simulink model "ReactionWheelPendulum"  (R2019b)
settings: Solver=FixedStepDiscrete  StartTime=0.0  StopTime=1  FixedStep=.005  RelTol=1e-3
values from neighbouring files (symbols this model uses):
  Bb = 0.0    [ReactionWheelPendulum.sldd]
  BodyCGDist_mm = 73.103937    [ReactionWheelPendulum.sldd]
  g_mps_2 = 9.81    [ReactionWheelPendulum.sldd]
  GearRatio_na = 3.0    [ReactionWheelPendulum.sldd]
  IBodyPivot_kgm_2 = 0.004054322    [ReactionWheelPendulum.sldd]
  IWheelCG_kgm_2 = 0.00010714633    [ReactionWheelPendulum.sldd]
  IWheelPivot_kgm_2 = 0.00054580359    [ReactionWheelPendulum.sldd]
  MassBody_kg = 0.49436    [ReactionWheelPendulum.sldd]
  MassWheel_kg = 0.092779    [ReactionWheelPendulum.sldd]
  WheelCGDist_mm = 68.760176    [ReactionWheelPendulum.sldd]
undefined symbols (not defined in the file or in its folder): DiscIntNeverNeededParam
libraries: simulink x6, simulink_extras x3
settings Model: DataDictionary=ReactionWheelPendulum.sldd  Creator=aloehr  LastModifiedBy=aloehr

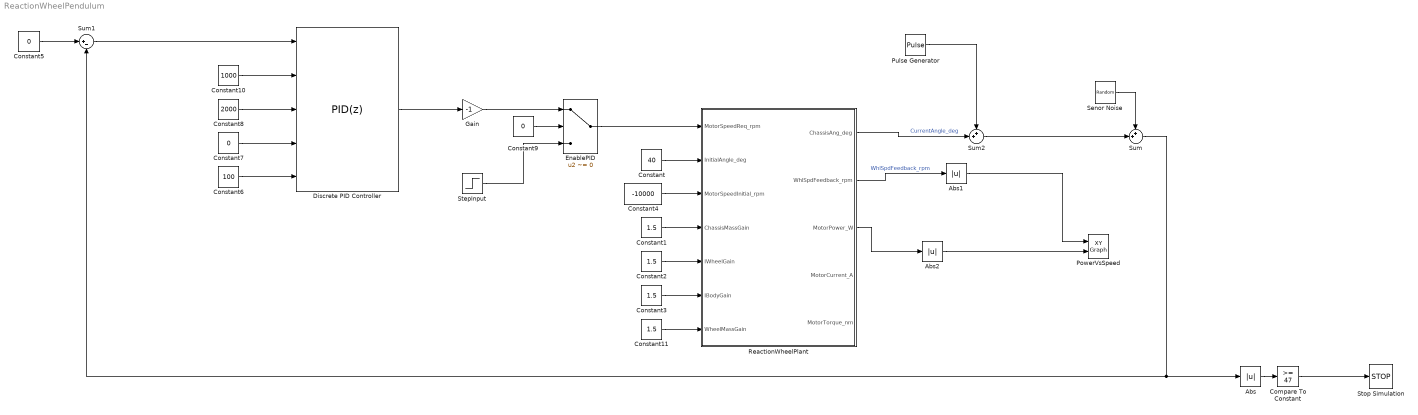
== system ReactionWheelPendulum ==
  Abs : Abs
  Abs1 : Abs
  Abs2 : Abs
  Compare To Constant : simulink/Logic and Bit Operations/Compare To Constant  relop=>=  const=47  OutDataTypeStr=boolean
  Constant : Constant  Value=40
  Constant{1..3,11} (4 alike) : Constant  Value=1.5
  Constant10 : Constant  Value=1000
  Constant4 : Constant  Value=-10000
  Constant5 : Constant  Value=0
  Constant6 : Constant  Value=100
  Constant7 : Constant  Value=0
  Constant8 : Constant  Value=2000
  Constant9 : Constant  Value=0
  Discrete PID Controller : simulink/Continuous/PID Controller  Controller=PID  Form=Parallel  TimeDomain=Discrete-time  SampleTime=-1  IntegratorMethod=Forward Euler  FilterMethod=Forward Euler  ControllerParametersSource=external  P=1  I=1  D=0  UseFilter=on  N=100  TunerSelectOption=Transfer Function Based (PID Tuner App)  InitialConditionSource=internal  InitialConditionForIntegrator=0  InitialConditionForFilter=0  DifferentiatorICPrevScaledInput=0  ExternalReset=none  TrackingMode=off  Kt=1  LimitOutput=on  UpperSaturationLimit=11000  LowerSaturationLimit=-11000  LinearizeAsGain=off  AntiWindupMode=none  Kb=1  POutMin=[]  POutMax=[]  IOutMin=[]  IOutMax=[]  DOutMin=[]  DOutMax=[]  NOutMin=[]  NOutMax=[]  SumOutMin=[]  SumOutMax=[]  SaturationOutMin=[]  SaturationOutMax=[]  PParamMin=[]  PParamMax=[]  IParamMin=[]  IParamMax=[]  DParamMin=[]  DParamMax=[]  NParamMin=[]  NParamMax=[]  KbParamMin=[]  KbParamMax=[]  KtParamMin=[]  KtParamMax=[]  KbOutMin=[]  KbOutMax=[]  KtOutMin=[]  KtOutMax=[]  IntegratorOutMin=[]  IntegratorOutMax=[]  FilterOutMin=[]  FilterOutMax=[]  SumI1OutMin=[]  SumI1OutMax=[]  SumI2OutMin=[]  SumI2OutMax=[]  SumI3OutMin=[]  SumI3OutMax=[]  SumI4OutMin=[]  SumI4OutMax=[]  SumDOutMin=[]  SumDOutMax=[]  DifferentiatorOutMin=[]  DifferentiatorOutMax=[]  FilterDiffOutCoefMin=[]  FilterDiffOutCoefMax=[]  ReciprocalOutMin=[]  ReciprocalOutMax=[]  SumDenOutMin=[]  SumDenOutMax=[]  SumNumOutMin=[]  SumNumOutMax=[]  DivideOutMin=[]  DivideOutMax=[]  IntegratorContinuousStateAttributes=''  IntegratorStateMustResolveToSignalObject=off  IntegratorRTWStateStorageClass=Auto  FilterContinuousStateAttributes=''  FilterStateMustResolveToSignalObject=off  FilterRTWStateStorageClass=Auto  ParallelPVariant=ExternalParameters  IdealPVariant=Disabled  IVariant=ExternalParameters  DVariant=ExternalParameters  IntegratorVariant=Discrete  SatVariant=Enabled  AWVariant=Passthrough  PCopyVariant=Disabled  TRVariant=Disabled  FdbkBlocksVariant=Forward  IdealPFdbkVariant=Disabled  SatFdbkVariant=Disabled  DerivativeFilterVariant=ForwardEulerFilter  NVariant=ExternalParameters  NCopyVariant=Disabled  FilterICVariant=InternalICsFilter  IntegratorICVariant=InternalICs  ExternalResetVariant=Disabled  TRSumVariant=Passthrough  SumFdbkVariant=Disabled  SumVariant=Sum_PID
  EnablePID : Switch  Criteria=u2 ~= 0
  Gain : Gain  Gain=-1
  PowerVsSpeed : simulink/Sinks/XY Graph  xmin=0  xmax=11000  ymin=0  ymax=300  st=-1
  Pulse Generator : DiscretePulseGenerator  PulseType=Time based  Amplitude=5  Period=3  PulseWidth=10  PhaseDelay=1
  ReactionWheelPlant : Subsystem
  Senor Noise : UniformRandomNumber  Minimum=-.1  Maximum=.1  SampleTime=0.1
  StepInput : Step  Time=.015  Before=-10000  After=11000  SampleTime=0
  Stop Simulation : Stop
  Sum : Sum  Inputs=++|
  Sum1 : Sum  Inputs=|+-
  Sum2 : Sum  Inputs=++|
  wires:
  Constant/1 -> ReactionWheelPlant/2(InitialAngle_deg)
  Constant1/1 -> ReactionWheelPlant/4(ChassisMassGain)
  Constant2/1 -> ReactionWheelPlant/5(IWheelGain)
  Constant3/1 -> ReactionWheelPlant/6(IBodyGain)
  Senor Noise/1 -> Sum/1
  Sum/1 -> Sum1/2, Abs/1
  Constant5/1 -> Sum1/1
  Sum1/1 -> Discrete PID Controller/1
  Discrete PID Controller/1 -> Gain/1
  Constant6/1 -> Discrete PID Controller/5
  Constant7/1 -> Discrete PID Controller/4
  Constant8/1 -> Discrete PID Controller/3
  Compare To Constant/1 -> Stop Simulation/1
  Constant10/1 -> Discrete PID Controller/2
  Gain/1 -> EnablePID/1
  EnablePID/1 -> ReactionWheelPlant/1(MotorSpeedReq_rpm)
  Abs/1 -> Compare To Constant/1
  ReactionWheelPlant/3(MotorPower_W) -> Abs2/1
  ReactionWheelPlant/2(WhlSpdFeedback_rpm) -> Abs1/1  "WhlSpdFeedback_rpm"
  Abs1/1 -> PowerVsSpeed/1
  Abs2/1 -> PowerVsSpeed/2
  Constant9/1 -> EnablePID/2
  StepInput/1 -> EnablePID/3
  ReactionWheelPlant/1(ChassisAng_deg) -> Sum2/2  "CurrentAngle_deg"
  Sum2/1 -> Sum/2
  Constant11/1 -> ReactionWheelPlant/7(WheelMassGain)
  Pulse Generator/1 -> Sum2/1
  Constant4/1 -> ReactionWheelPlant/3(MotorSpeedInitial_rpm)

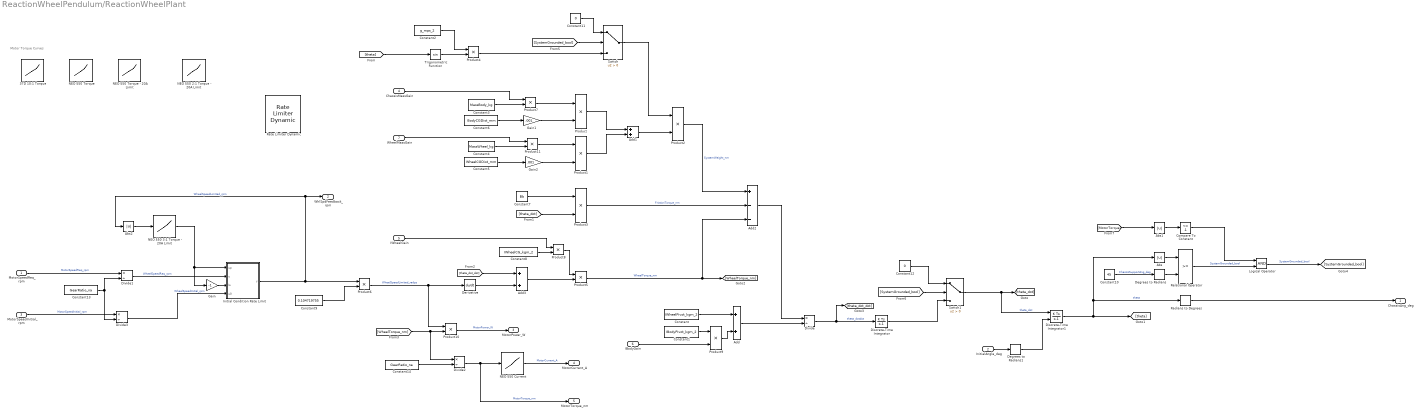
== system ReactionWheelPendulum/ReactionWheelPlant ==
  note: Motor Torque Curves
  MotorSpeedReq_rpm : Inport
  InitialAngle_deg : Inport  Port=2
  MotorSpeedInitial_rpm : Inport  Port=3
  ChassisMassGain : Inport  Port=4
  IWheelGain : Inport  Port=5
  IBodyGain : Inport  Port=6
  WheelMassGain : Inport  Port=7
  37D 10:1 Torque : Lookup_n-D  NumberOfTableDimensions=1  BreakpointsForDimension1=[0,1000]  Table=[55800,0.001]  InternalRulePriority=Speed  RndMeth=Simplest  InputSameDT=on
  Abs : Abs
  Abs1 : Abs
  Abs2 : Abs
  Add : Sum
  Add1 : Sum
  Add2 : Sum  Inputs=+--
  Add3 : Sum
  Compare To Constant : simulink/Logic and Bit Operations/Compare To Constant  relop=<=  const=.1  OutDataTypeStr=boolean
  Constant : Constant  Value=IWheelPivot_kgm_2  VectorParams1D=off
  Constant1 : Constant  Value=IBodyPivot_kgm_2
  Constant10 : Constant  Value=45
  Constant11 : Constant  Value=0
  Constant12 : Constant  Value=0
  Constant13 : Constant  Value=GearRatio_na
  Constant14 : Constant  Value=GearRatio_na
  Constant2 : Constant  Value=g_mps_2
  Constant3 : Constant  Value=MassBody_kg
  Constant4 : Constant  Value=MassWheel_kg
  Constant5 : Constant  Value=WheelCGDist_mm
  Constant6 : Constant  Value=BodyCGDist_mm
  Constant7 : Constant  Value=Bb
  Constant8 : Constant  Value=IWheelCG_kgm_2
  Constant9 : Constant  Value=0.104719755
  Degrees to Radians : simulink_extras/Transformations/Degrees to Radians
  Degrees to Radians1 : simulink_extras/Transformations/Degrees to Radians
  Derivative : Derivative
  Discrete-Time Integrator : DiscreteIntegrator  SampleTime=-1  ICPrevOutput=DiscIntNeverNeededParam  ICPrevScaledInput=DiscIntNeverNeededParam
  Discrete-Time Integrator1 : DiscreteIntegrator  InitialConditionSource=external  SampleTime=-1  ICPrevOutput=DiscIntNeverNeededParam  ICPrevScaledInput=DiscIntNeverNeededParam
  Divide{,1..3} (4 alike) : Product  Inputs=*/
  Gain : Gain  Gain=-1
  Gain1 : Gain  Gain=.001
  Gain2 : Gain  Gain=.001
  Initial Condition Rate Limit : Subsystem
  Logical Operator : Logic  AllPortsSameDT=off  OutDataTypeStr=boolean
  NEO 550 2:1 Torque - 20A Limit : Lookup_n-D  NumberOfTableDimensions=1  BreakpointsForDimension1=[0,4500,5500]  Table=[35000,35000,0]  InternalRulePriority=Speed  RndMeth=Simplest  InputSameDT=on
  NEO 550 3:1 Torque - 20A Limit : Lookup_n-D  NumberOfTableDimensions=1  BreakpointsForDimension1=[0,3000,3666.667]  Table=[35000,35000,0]  InternalRulePriority=Speed  RndMeth=Simplest  InputSameDT=on
  NEO 550 Current : Lookup_n-D  NumberOfTableDimensions=1  BreakpointsForDimension1=[0,.97]  Table=[0,100]  InternalRulePriority=Speed  RndMeth=Simplest  InputSameDT=on
  NEO 550 Torque : Lookup_n-D  NumberOfTableDimensions=1  BreakpointsForDimension1=[0,11000]  Table=[88300,0]  InternalRulePriority=Speed  RndMeth=Simplest  InputSameDT=on
  NEO 550 Torque - 20A Limit : Lookup_n-D  NumberOfTableDimensions=1  BreakpointsForDimension1=[0,9000,11000]  Table=[17500,17500,0]  InternalRulePriority=Speed  RndMeth=Simplest  InputSameDT=on
  Product{,1..11} (12 alike) : Product
  Radians to Degrees : simulink_extras/Transformations/Radians to Degrees
  Rate Limiter Dynamic : simulink/Discontinuities/Rate Limiter Dynamic
      settings: SourceProductName=Simulink
  Relational Operator : RelationalOperator  OutDataTypeStr=boolean  RndMeth=Simplest
  Switch : Switch  Criteria=u2 > Threshold
  Switch1 : Switch  Criteria=u2 > Threshold
  Trigonometric Function : Trigonometry
  ChassisAng_deg : Outport
  WhlSpdFeedback_rpm : Outport  Port=2
  MotorPower_W : Outport  Port=3
  MotorCurrent_A : Outport  Port=4
  MotorTorque_nm : Outport  Port=5
  wires:
  Product3/1 -> Add2/2  "FrictionTorque_nm"
  InitialAngle_deg/1 -> Degrees to Radians1/1
  Constant4/1 -> Product11/2
  Add1/1 -> Product2/2
  Product1/1 -> Add1/2
  Product2/1 -> Add2/1  "SystemWeight_nm"
  Add2/1 -> Divide/1
  Divide/1 -> Discrete-Time Integrator/1, [theta_dot_dot]  "theta_dotdot"
  Constant3/1 -> Product7/2
  Constant5/1 -> Gain2/1
  Product/1 -> Add1/1
  Add3/1 -> Product5/2
  Switch/1 -> Product2/1
  Constant7/1 -> Product3/1
  [theta_dot] -> Product3/2
  Add/1 -> Divide/2
  Constant6/1 -> Gain1/1
  Product8/1 -> Product5/1
  Derivative/1 -> Add3/2
  Constant/1 -> Add/1
  Constant1/1 -> Product9/1
  Constant9/1 -> Product6/2
  Degrees to Radians1/1 -> Discrete-Time Integrator1/2
  Radians to Degrees/1 -> ChassisAng_deg/1
  Discrete-Time Integrator1/1 -> [theta], Radians to Degrees/1, Abs/1  "theta"
  Constant10/1 -> Degrees to Radians/1  "ChassisSupportAng_deg"
  Degrees to Radians/1 -> Relational Operator/2
  Gain1/1 -> Product/2
  Gain2/1 -> Product1/2
  Constant2/1 -> Product4/1
  [theta] -> Trigonometric Function/1
  Trigonometric Function/1 -> Product4/2
  Product4/1 -> Switch/3
  Abs/1 -> Relational Operator/1
  Logical Operator/1 -> [SystemGrounded_bool]  "SystemGrounded_bool"
  [SystemGrounded_bool] -> Switch/2
  Constant11/1 -> Switch/1
  Discrete-Time Integrator/1 -> Switch1/3
  Switch1/1 -> Discrete-Time Integrator1/1, [theta_dot]  "theta_dot"
  [SystemGrounded_bool] -> Switch1/2
  Constant12/1 -> Switch1/1
  Abs1/1 -> Compare To Constant/1
  Relational Operator/1 -> Logical Operator/2  "SystemGrounded_bool"
  Compare To Constant/1 -> Logical Operator/1
  Product5/1 -> [WheelTorque_nm], Add2/3  "WheelTorque_nm"
  [MotorTorque] -> Abs1/1
  Product6/1 -> Derivative/1, Product10/1  "WheelSpeedLimited_radps"
  Initial Condition Rate Limit/1(Y) -> Abs2/1, WhlSpdFeedback_rpm/1, Product6/1  "WheelSpeedLimited_rpm"
  Product7/1 -> Product/1
  ChassisMassGain/1 -> Product7/1
  Constant8/1 -> Product8/2
  IWheelGain/1 -> Product8/1
  [theta_dot_dot] -> Add3/1
  Product9/1 -> Add/2
  IBodyGain/1 -> Product9/2
  NEO 550 3:1 Torque - 20A Limit/1 -> Gain/1, Initial Condition Rate Limit/1(up)
  Gain/1 -> Initial Condition Rate Limit/3(lo)
  [WheelTorque_nm] -> Divide2/1, Product10/2
  Product10/1 -> MotorPower_W/1  "MotorPower_W"
  Abs2/1 -> NEO 550 3:1 Torque - 20A Limit/1
  NEO 550 Current/1 -> MotorCurrent_A/1  "MotorCurrent_A"
  MotorSpeedReq_rpm/1 -> Divide1/1  "MotorSpeedReq_rpm"
  Divide1/1 -> Initial Condition Rate Limit/2(u)  "WheelSpeedReq_rpm"
  Constant13/1 -> Divide1/2, Divide3/2
  Constant14/1 -> Divide2/2
  Divide2/1 -> MotorTorque_nm/1, NEO 550 Current/1  "MotorTorque_nm"
  Product11/1 -> Product1/1
  WheelMassGain/1 -> Product11/1
  MotorSpeedInitial_rpm/1 -> Divide3/1  "MotorSpeedInitial_rpm"
  Divide3/1 -> Initial Condition Rate Limit/4(u0)  "WheelSpeedInitial_rpm"

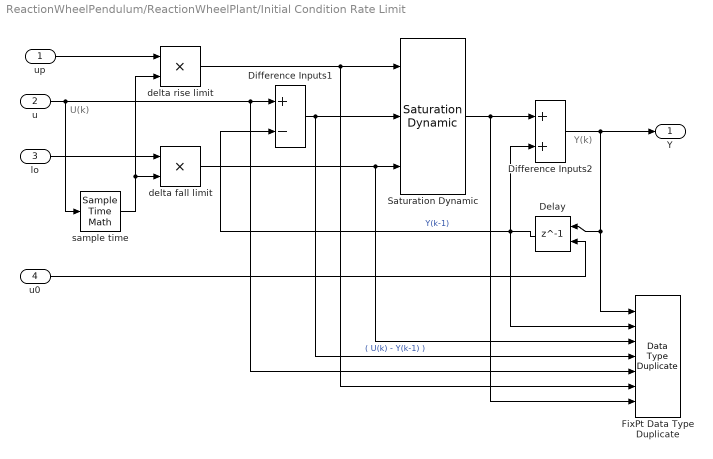
== system ReactionWheelPendulum/ReactionWheelPlant/Initial Condition Rate Limit ==
  note: U(k)
  note: Y(k)
  up : Inport
  u : Inport  Port=2
  lo : Inport  Port=3
  u0 : Inport  Port=4
  Delay : Delay  DelayLength=1  InitialConditionSource=Input port  InitialCondition=-3333
      settings: InputPortMap=u0,p4
  Difference Inputs1 : Sum  Description=Add in CPU  DisableCoverage=on  Inputs=+-  OutDataTypeStr=Inherit: Inherit via back propagation
  Difference Inputs2 : Sum  Description=Add in CPU  OutDataTypeStr=Inherit: Inherit via back propagation
  FixPt Data Type Duplicate : DataTypeDuplicate  DisableCoverage=on  NumInputPorts=7
  Saturation Dynamic : simulink/Discontinuities/Saturation Dynamic  OutMin=[]  OutMax=[]  OutDataTypeStr=Inherit: Same as second input  OutDataType=fixdt(1, 16)  OutScaling=2^-10  DoSatur=off
  delta fall limit : Product  DisableCoverage=on  Inputs=**  OutDataTypeStr=Inherit: Inherit via back propagation  SaturateOnIntegerOverflow=on
  delta rise limit : Product  DisableCoverage=on  Inputs=**  OutDataTypeStr=Inherit: Inherit via back propagation  SaturateOnIntegerOverflow=on
  sample time : SampleTimeMath  DisableCoverage=on  TsampMathOp=Ts Only  weightValue=1
  Y : Outport  InitialOutput=0
  wires:
  lo/1 -> delta fall limit/1
  delta rise limit/1 -> FixPt Data Type Duplicate/6, Saturation Dynamic/1
  up/1 -> delta rise limit/1
  u/1 -> Difference Inputs1/1, FixPt Data Type Duplicate/5, sample time/1
  sample time/1 -> delta fall limit/2, delta rise limit/2
  Saturation Dynamic/1 -> Difference Inputs2/1, FixPt Data Type Duplicate/7
  Delay/1 -> Difference Inputs1/2, FixPt Data Type Duplicate/2, Difference Inputs2/2  "Y(k-1)"
  Difference Inputs1/1 -> FixPt Data Type Duplicate/4, Saturation Dynamic/2  "( U(k) - Y(k-1) )"
  Difference Inputs2/1 -> Y/1, Delay/1, FixPt Data Type Duplicate/1
  delta fall limit/1 -> FixPt Data Type Duplicate/3, Saturation Dynamic/3
  u0/1 -> Delay/2
